simulink model "equations"  (R2020a)
settings: Solver=VariableStepAuto  StartTime=0.0  StopTime=10.0  RelTol=1e-3
settings Model: Creator=ILIA  LastModifiedBy=ILIA

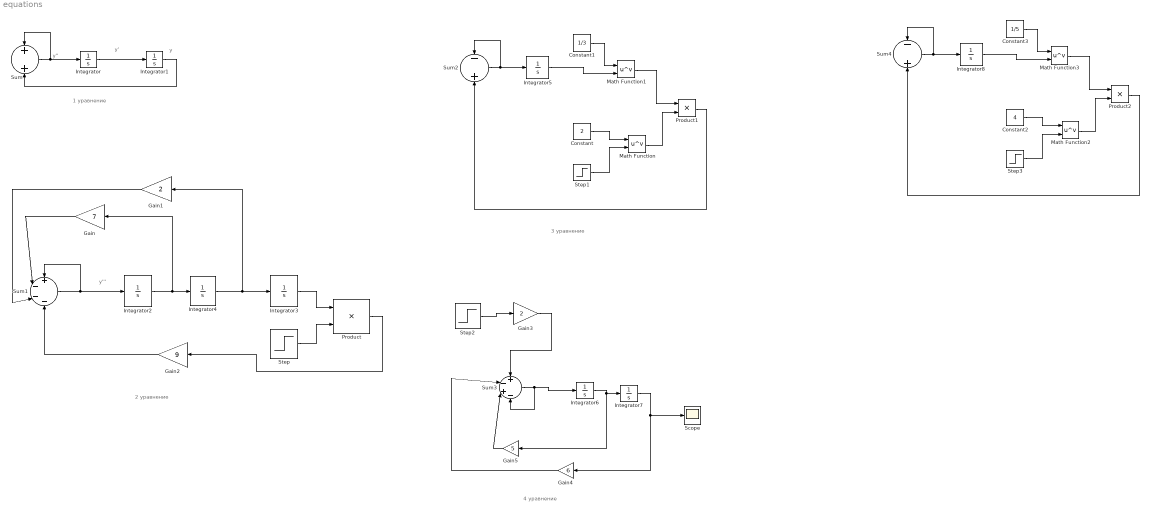
== system equations ==
  note: 4 уравнение
  note: 3 уравнение
  note: 2 уравнение
  note: 1 уравнение
  note: y'''
  note: y''
  note: y'
  note: y
  Constant : Constant  Value=2
  Constant1 : Constant  Value=1/3
  Constant2 : Constant  Value=4
  Constant3 : Constant  Value=1/5
  Gain : Gain  Gain=7
  Gain1 : Gain  Gain=2
  Gain2 : Gain  Gain=9
  Gain3 : Gain  Gain=2
  Gain4 : Gain  Gain=6
  Gain5 : Gain  Gain=5
  Integrator{,1..8} (9 alike) : Integrator
  Math Function{,1..3} (4 alike) : Math  Operator=pow  SaturateOnIntegerOverflow=on
  Product : Product
  Product1 : Product
  Product2 : Product
  Scope : Scope
  Step{,1..3} (4 alike) : Step  SampleTime=0
  Sum : Sum
  Sum1 : Sum  Inputs=+---
  Sum2 : Sum  Inputs=-+
  Sum3 : Sum  Inputs=+-+-
  Sum4 : Sum  Inputs=-+
  wires:
  Integrator/1 -> Integrator1/1
  Integrator1/1 -> Sum/2
  Sum/1 -> Sum/1, Integrator/1
  Integrator4/1 -> Gain1/1, Integrator3/1
  Sum1/1 -> Sum1/1, Integrator2/1
  Integrator2/1 -> Gain/1, Integrator4/1
  Gain/1 -> Sum1/2
  Gain1/1 -> Sum1/3
  Step/1 -> Product/2
  Integrator3/1 -> Product/1
  Product/1 -> Gain2/1
  Gain2/1 -> Sum1/4
  Sum2/1 -> Sum2/1, Integrator5/1
  Integrator5/1 -> Math Function1/2
  Constant1/1 -> Math Function1/1
  Math Function1/1 -> Product1/1
  Constant/1 -> Math Function/1
  Step1/1 -> Math Function/2
  Math Function/1 -> Product1/2
  Product1/1 -> Sum2/2
  Step2/1 -> Gain3/1
  Gain3/1 -> Sum3/1
  Sum3/1 -> Sum3/4, Integrator6/1
  Integrator6/1 -> Gain5/1, Integrator7/1
  Integrator7/1 -> Scope/1, Gain4/1
  Gain4/1 -> Sum3/2
  Gain5/1 -> Sum3/3
  Integrator8/1 -> Math Function3/2
  Constant3/1 -> Math Function3/1
  Product2/1 -> Sum4/2
  Step3/1 -> Math Function2/2
  Math Function3/1 -> Product2/1
  Constant2/1 -> Math Function2/1
  Math Function2/1 -> Product2/2
  Sum4/1 -> Sum4/1, Integrator8/1
